simulink model "HDLDecimator"  (R2024a)
settings: Solver=FixedStepDiscrete  StartTime=0.0  StopTime=stopTime  RelTol=1e-3
values from neighbouring files (symbols this model uses):
  fIn = CONST.fADC    [testDecimator.m]
  fOut = fIn/CONST.rxM    [testDecimator.m]
libraries: dspsrcs4 x2, HDL_ieee_8021513 x2, whdlutilities x1
settings Model: DataTypeOverride=Off  Creator=cotti  LastModifiedBy=cotti
settings OptimizationCC: BlockReduction=off  ConditionallyExecuteInputs=off  DefaultParameterBehavior=Inlined  InheritOutputTypeSmallerThanSingle=on
settings DebuggingCC: AlgebraicLoopMsg=error  ArtificialAlgebraicLoopMsg=error  SingleTaskRateTransMsg=error  UnconnectedInputMsg=warning  UnconnectedOutputMsg=warning  UnconnectedLineMsg=warning
settings HardwareCC: ProdBitPerPointer=32  ProdBitPerSizeT=32  ProdBitPerPtrDiffT=32  ProdLargestAtomicFloat=None  ProdIntDivRoundTo=Undefined  ProdEndianess=Unspecified  ProdWordSize=32  ProdHWDeviceType=ASIC/FPGA->ASIC/FPGA  TargetBitPerLong=64  TargetBitPerPointer=64  TargetBitPerSizeT=64  TargetBitPerPtrDiffT=64  TargetLongLongMode=on  TargetIntDivRoundTo=Zero  TargetEndianess=LittleEndian  TargetWordSize=64  TargetHWDeviceType=Custom Processor->MATLAB Host Computer  ProdEqTarget=off

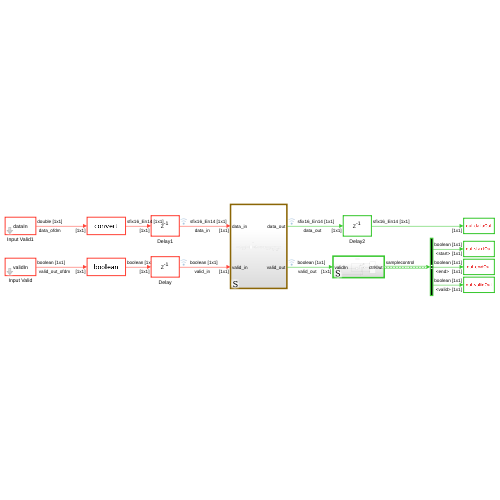
[thumbnail: Simulink's stored preview of the top-level diagram]
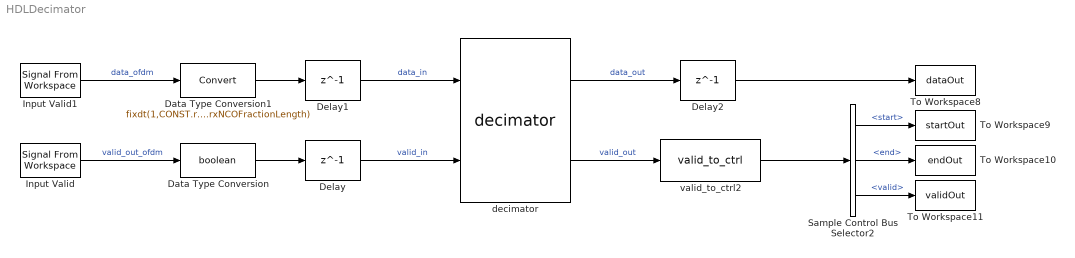
== system HDLDecimator ==
  Data Type Conversion : DataTypeConversion  OutDataTypeStr=boolean  SaturateOnIntegerOverflow=off  RndMeth=Floor
  Data Type Conversion1 : DataTypeConversion  OutDataTypeStr=fixdt(1,CONST.rxNCOWordLength,CONST.rxNCOFractionLength)  SaturateOnIntegerOverflow=off  RndMeth=Floor
  Delay : Delay  DelayLength=1  InitialCondition=0  UseCircularBuffer=on
  Delay1 : Delay  DelayLength=1  InitialCondition=0  UseCircularBuffer=on
  Delay2 : Delay  DelayLength=1  InitialCondition=0  UseCircularBuffer=on
  Input Valid : dspsrcs4/Signal From Workspace  X=validIn  Ts=1/fIn  nsamps=1  OutputAfterFinalValue=Setting to zero  ignoreOrWarnInputAndFrameLengths=off  OutputFrames=off
  Input Valid1 : dspsrcs4/Signal From Workspace  X=dataIn  Ts=1/fIn  nsamps=1  OutputAfterFinalValue=Setting to zero  ignoreOrWarnInputAndFrameLengths=off  OutputFrames=off
  Sample Control Bus Selector2 : whdlutilities/Sample Control Bus Selector  OutputSignals=start,end,valid
  To Workspace10 : ToWorkspace  VariableName=endOut  SampleTime=1/fOut
      settings: Save2DSignal=2-D array (concatenate along first dimension)
  To Workspace11 : ToWorkspace  VariableName=validOut  SampleTime=1/fOut
      settings: Save2DSignal=2-D array (concatenate along first dimension)
  To Workspace8 : ToWorkspace  VariableName=dataOut  SampleTime=1/fOut
      settings: Save2DSignal=2-D array (concatenate along first dimension)
  To Workspace9 : ToWorkspace  VariableName=startOut  SampleTime=1/fOut
      settings: Save2DSignal=2-D array (concatenate along first dimension)
  decimator : HDL_ieee_8021513/decimator  SystemSampleTime=-1  VariantActivationTime=update diagram  AllowFlexibleInterface=on  Latency=0  AutoFrameSizeCalculation=off
      settings: SourceProductName=HDL IEEE 8021513
  valid_to_ctrl2 : HDL_ieee_8021513/valid_to_ctrl  SystemSampleTime=-1  VariantActivationTime=update diagram  AllowFlexibleInterface=on  Latency=0  AutoFrameSizeCalculation=off
      settings: SourceProductName=HDL IEEE 8021513
  wires:
  Sample Control Bus Selector2/3 -> To Workspace11/1  "<valid>"
  Sample Control Bus Selector2/1 -> To Workspace9/1  "<start>"
  valid_to_ctrl2/1 -> Sample Control Bus Selector2/1
  Sample Control Bus Selector2/2 -> To Workspace10/1  "<end>"
  Delay2/1 -> To Workspace8/1
  Input Valid1/1 -> Data Type Conversion1/1  "data_ofdm"
  Input Valid/1 -> Data Type Conversion/1  "valid_out_ofdm"
  decimator/1 -> Delay2/1  "data_out"
  decimator/2 -> valid_to_ctrl2/1  "valid_out"
  Data Type Conversion/1 -> Delay/1
  Data Type Conversion1/1 -> Delay1/1
  Delay/1 -> decimator/2  "valid_in"
  Delay1/1 -> decimator/1  "data_in"
